simulink model "LinThermo"  (Simulink 7.9)
settings: Solver=ode45  StartTime=0.0  StopTime=10.0  FixedStep=0.01  RelTol=1e-3
settings Model: Creator=Karthik Manamcheri  LastModifiedBy=parasara
settings DebuggingCC: FcnCallInpInsideContextMsg=Use local settings  StrictBusMsg=Warning
settings GRTTargetCC: CombineOutputUpdateFcns=off  GRTInterface=on

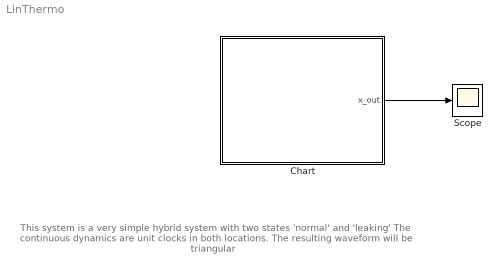
== system LinThermo ==
  note: This system is a very simple hybrid system with two states 'normal'
      | and 'leaking'
      | The continuous dynamics are unit clocks in both locations.
      | The resulting waveform will be triangular
  Chart : Stateflow chart  TreatAsAtomicUnit=on
  Scope : Scope
  wires:
  Chart/1(x_out) -> Scope/1

== stateflow chart Chart ==
  settings: updateMethod=CONTINUOUS
  state heating
    du:
    x_dot = 40 - 0.5*x;
    x_out = x;
  state cooling
    du:
    x_dot = 30 -0.5*x;
    x_out = x;
  note: @annotation-mode=heating;
      | k=1;
      | gamma=-0.1;
  note: @annotation-mode=cooling;
      | k=1;
      | gamma=-0.1;
  heating -> cooling : [x >= 75]
  cooling -> heating : [x <= 65]
  (default) -> heating : {x = 70}
  data: x local double; x_out output double
  data x settings: updateMethod=SF_CONTINUOUS_TIME_DATA
